simulink model "dpsk_Simulink"  (R2020b)
settings: Solver=FixedStepAuto  StartTime=0.0  StopTime=stopTime  FixedStep=stepSize  RelTol=1e-3
values from neighbouring files (symbols this model uses):
  angleConstel = angle(phaseConstel)    [dpsk_parameters.m]
  M = 8    [dpsk_parameters.m]
  stepSize = 1    [dpsk_parameters.m]
libraries: commchan3 x1, commsink2 x1, commdigbbndpm3 x1, commrandsrc3 x1
settings Model: Creator=peytonaplin  LastModifiedBy=peytonaplin

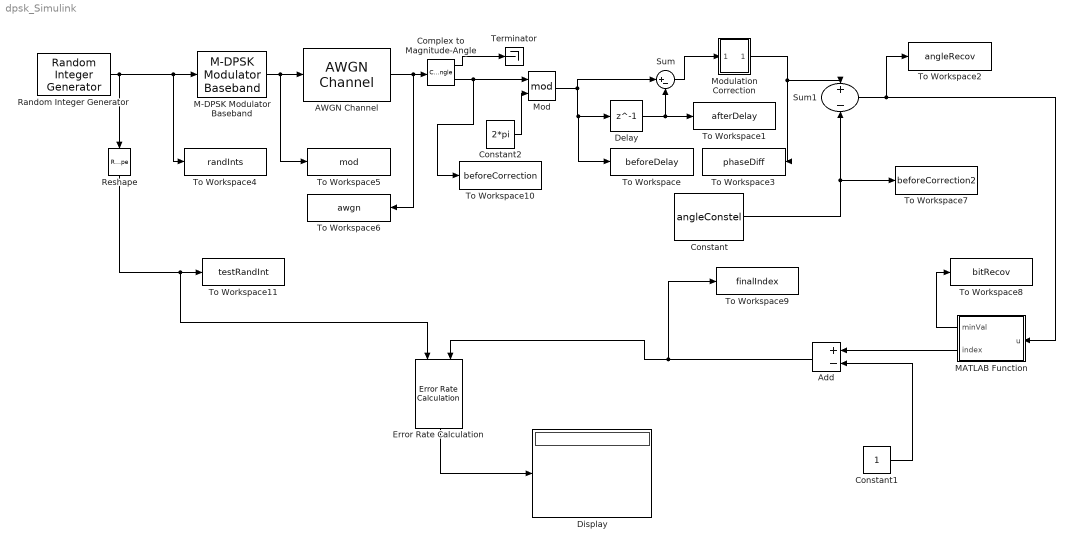
== system dpsk_Simulink ==
  AWGN Channel : commchan3/AWGN Channel  InputProcessing=Columns as channels (frame based)  seed=67  noiseMode="Signal to noise ratio  (Eb/No)"  EbNodB=snr  EsNodB=10  SNRdB=10  bitsPerSym=log2(M)  Ps=1  Tsym=1  variance=1
  Add : Sum  Inputs=+-
  Complex to Magnitude-Angle : ComplexToMagnitudeAngle
  Constant : Constant  Value=angleConstel
  Constant1 : Constant
  Constant2 : Constant  Value=2*pi
  Delay : Delay  DelayLength=1  InitialCondition=0
  Display : Display
  Error Rate Calculation : commsink2/Error Rate Calculation  N=0  st_delay=0  cp_mode=Entire frame  subframe=[]  PMode=Port  WsName=ErrorVec  RsMode2=off  stop=off  numErr=100  maxBits=1e6
      settings: SourceProductName=Communications Toolbox
  M-DPSK Modulator Baseband : commdigbbndpm3/M-DPSK Modulator Baseband  M=M  InType=Integer  Enc=Binary  Ph=phaseoffset  outDtype=double
      settings: SourceProductBaseCode=CM
  MATLAB Function : MATLAB Function  TreatAsAtomicUnit=on
  Mod : Math  Operator=mod  SaturateOnIntegerOverflow=on
  Modulation Correction : Subsystem
  Random Integer Generator : commrandsrc3/Random Integer Generator  SetSize=M  SeedSource=Auto  Seed=0  SampleTime=stepSize  SamplesPerFrame=samples  OutputDataType=double  SimulateUsing=Interpreted execution
  Reshape : Reshape
  Sum : Sum  Inputs=|+-
  Sum1 : Sum  Inputs=+-
  Terminator : Terminator
  To Workspace : ToWorkspace  VariableName=beforeDelay  SampleTime=-1
  To Workspace1 : ToWorkspace  VariableName=afterDelay  SampleTime=-1
  To Workspace10 : ToWorkspace  VariableName=beforeCorrection  SampleTime=-1
  To Workspace11 : ToWorkspace  VariableName=testRandInt  SampleTime=-1
  To Workspace2 : ToWorkspace  VariableName=angleRecov  SampleTime=-1
      settings: Save2DSignal=2-D array (concatenate along first dimension)
  To Workspace3 : ToWorkspace  VariableName=phaseDiff  SampleTime=-1
  To Workspace4 : ToWorkspace  VariableName=randInts  SampleTime=-1
  To Workspace5 : ToWorkspace  VariableName=mod  SampleTime=-1
  To Workspace6 : ToWorkspace  VariableName=awgn  SampleTime=-1
  To Workspace7 : ToWorkspace  VariableName=beforeCorrection2  SampleTime=-1
  To Workspace8 : ToWorkspace  VariableName=bitRecov  SampleTime=-1
      settings: Save2DSignal=2-D array (concatenate along first dimension)
  To Workspace9 : ToWorkspace  VariableName=finalIndex  SampleTime=-1
  wires:
  Random Integer Generator/1 -> Reshape/1, To Workspace4/1, M-DPSK Modulator Baseband/1
  M-DPSK Modulator Baseband/1 -> To Workspace5/1, AWGN Channel/1
  Complex to Magnitude-Angle/1 -> Terminator/1
  AWGN Channel/1 -> To Workspace6/1, Complex to Magnitude-Angle/1
  Complex to Magnitude-Angle/2 -> Mod/1, To Workspace10/1
  Sum/1 -> Modulation Correction/1(In1)
  Sum1/1 -> MATLAB Function/1(u), To Workspace2/1
  MATLAB Function/1(minVal) -> To Workspace8/1
  Delay/1 -> To Workspace1/1, Sum/2
  Mod/1 -> Sum/1, To Workspace/1, Delay/1
  Constant/1 -> Sum1/2, To Workspace7/1
  Modulation Correction/1(Out1) -> To Workspace3/1, Sum1/1
  Reshape/1 -> Error Rate Calculation/1, To Workspace11/1
  Error Rate Calculation/1 -> Display/1
  Constant2/1 -> Mod/2
  MATLAB Function/2(index) -> Add/1
  Constant1/1 -> Add/2
  Add/1 -> To Workspace9/1, Error Rate Calculation/2

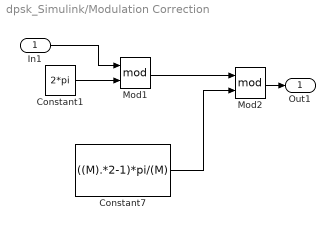
== system dpsk_Simulink/Modulation Correction ==
  In1 : Inport
  Constant1 : Constant  Value=2*pi
  Constant7 : Constant  Value=((M).*2-1)*pi/(M)
  Mod1 : Math  Operator=mod  SaturateOnIntegerOverflow=on
  Mod2 : Math  Operator=mod  SaturateOnIntegerOverflow=on
  Out1 : Outport
  wires:
  Constant7/1 -> Mod2/2
  Constant1/1 -> Mod1/2
  Mod1/1 -> Mod2/1
  In1/1 -> Mod1/1
  Mod2/1 -> Out1/1

== matlab function dpsk_Simulink/MATLAB Function ==
  data: u input; minVal output; index output
function [minVal, index] = fcn(u)

[minVal, index] = min(abs(u));
